simulink model "rebi"  (R2026a)
settings: Solver=ode1  StopTime=40  FixedStep=0.001  EnableMultiTasking=on
PostLoadFcn:
  | , if any(exist('dsrtsu_mdlpostloadfcn', 'file') == [2, 3, 6]), try dsrtsu_mdlpostloadfcn('Execute', bdroot); catch fprintf('Error in PostLoadFcn (dsrtsu_mdlpostloadfcn) for model "%s":\n %s\n', bdroot, lasterr); end, end,
values from neighbouring files (symbols this model uses):
  A = [0 1 ; -w0^2 -2*xhi*w0]    [integral_state_feedback_pole_placement.m]    (also in lqr_integral_control.m = [-2*xhi*omega0  -omega0^2  0     0           0)
  B = [0 ; k*w0]    [integral_state_feedback_pole_placement.m]    (also in lqr_integral_control.m = [Ke*omega0^2     Ke*omega0^2)
  C = [1 0]    [integral_state_feedback_pole_placement.m]    (also in lqr_integral_control.m = [0 1 0 0 0)
  Ki = K(:, n+1:n+p)    [lqr_integral_control.m]
  Kp = K(:, 1:n)    [lqr_integral_control.m]
settings Model: DSRTSU_INTERNAL_RTI_VER=370  DSRTSU_INTERNAL_RTI_TYPE=rti1104  Creator=eleve  LastModifiedBy=DevKumar
settings DataIOCC: SignalLoggingSaveFormat=ModelDataLogs
settings OptimizationCC: OptimizeBlockIOStorage=off  BufferReuse=off  ExpressionFolding=off  LocalBlockOutputs=off
settings DebuggingCC: UnderspecifiedInitializationDetection=Classic
settings HardwareCC: ProdEndianess=BigEndian  ProdHWDeviceType=Generic->Custom  TargetIntDivRoundTo=Zero  TargetEndianess=BigEndian  TargetHWDeviceType=Generic->Custom
settings RTWCC: SystemTargetFile=rti1104.tlc  MakeCommand=make_rti  TemplateMakefile=rti1104.tmf  Description=dSPACE DS1104 Hardware Platform
settings STFCustomTargetCC: SystemTargetFile=rti1104.tlc  MultiwordLength=2048.0  ParMdlRefBuildCompliant=on  CPPClassGenCompliant=on  TimeScaleFactorNonUI=OPTION_DISABLED  TimeScaleFactor=1.0  CCompilerOptimizationOptsPopup_=Default  ExecutionModeNonUI=RTSIM  TAStimulusEngineEnable=off  InitialSimState=RUN  AllowReservedHostServiceNums=off  ExecutionMode=real-time  AssertionMode=OFF  LoadAfterBuild=on  CCompilerEffectiveOptimizationOpts=-Ot -Oi -Or -Ox -D_INLINE  CCompilerOptimizationOptsNonUI=USE_DEFAULT  BoardNameNonUI=OPTION_DISABLED  LoadToFlash=off  TRCGenerateParamValues=off  LoadApplNonUI=ON  TRCApplySubsystemPermissions=off  PlatformSelectionPopup=Auto  TRCMaskParameters=off  TRCGenerateStates=off  TRCOnlyGlobals=off  TRCGenerateDerivatives=off  TRCGenerateLabels=on  TRCIsOmitVdOn=off  TRCGenerateVirtualBlocks=on
settings GRTTargetCC: ExtModeMexFile=noextcomm  CompOptLevelCompliant=off  ConcurrentExecutionCompliant=off  CombineOutputUpdateFcns=off  MatFileLogging=off  GRTInterface=on

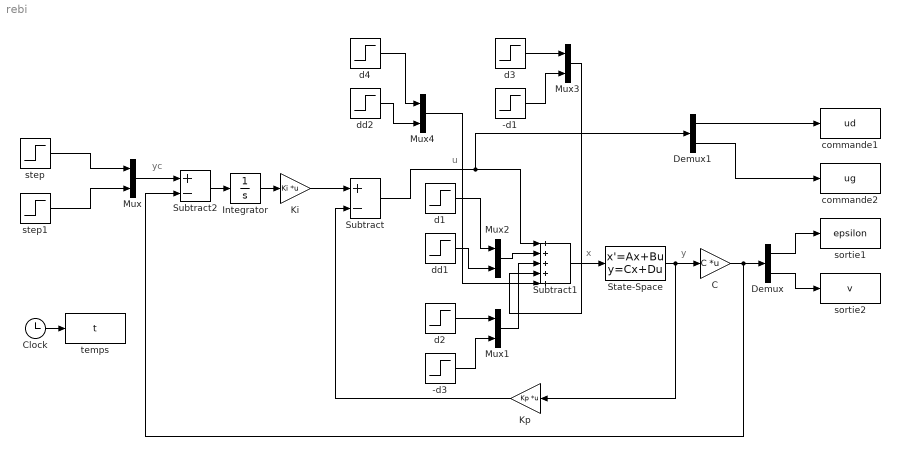
== system rebi ==
  note: u
  note: yc
  note: x
  note: y
  -d1 : Step  Time=11  FinalValue=5  SampleTime=0
  -d3 : Step  Time=10  FinalValue=-5  SampleTime=0
  C : Gain  Gain=C  Multiplication=Matrix(K*u) (u vector)
  Clock : Clock
  Demux : Demux  Outputs=2
  Demux1 : Demux  Outputs=2
  Integrator : Integrator
  Ki : Gain  Gain=Ki  Multiplication=Matrix(K*u) (u vector)
  Kp : Gain  Gain=Kp  Multiplication=Matrix(K*u) (u vector)
  Mux{,1..4} (5 alike) : Mux  Inputs=2
  State-Space : StateSpace  A=A  B=B  C=eye(5)  D=zeros(5,2)  InitialCondition=0
  Subtract : Sum  Inputs=+-
  Subtract1 : Sum  Inputs=+++++
  Subtract2 : Sum  Inputs=+-
  commande1 : ToWorkspace  VariableName=ud  SampleTime=-1
  commande2 : ToWorkspace  VariableName=ug  SampleTime=-1
  d1 : Step  Time=10  FinalValue=5  SampleTime=0
  d2 : Step  Time=10  FinalValue=5  SampleTime=0
  d3 : Step  Time=11  FinalValue=-5  SampleTime=0
  d4 : Step  Time=11  FinalValue=5  SampleTime=0
  dd1 : Step  Time=10  FinalValue=5  SampleTime=0
  dd2 : Step  Time=11  FinalValue=5  SampleTime=0
  sortie1 : ToWorkspace  VariableName=epsilon  SampleTime=-1
  sortie2 : ToWorkspace  VariableName=v  SampleTime=-1
  step : Step  FinalValue=pi/6  SampleTime=0
  step1 : Step  SampleTime=0
  temps : ToWorkspace  VariableName=t  SampleTime=-1
  wires:
  Subtract2/1 -> Integrator/1
  Integrator/1 -> Ki/1
  Ki/1 -> Subtract/1
  Kp/1 -> Subtract/2
  Subtract/1 -> Subtract1/1, Demux1/1
  State-Space/1 -> C/1, Kp/1
  Clock/1 -> temps/1
  C/1 -> Demux/1, Subtract2/2
  Demux/1 -> sortie1/1
  Demux/2 -> sortie2/1
  Demux1/1 -> commande1/1
  Demux1/2 -> commande2/1
  step/1 -> Mux/1
  step1/1 -> Mux/2
  Mux/1 -> Subtract2/1
  Subtract1/1 -> State-Space/1
  d1/1 -> Mux2/1
  dd1/1 -> Mux2/2
  Mux2/1 -> Subtract1/2
  d2/1 -> Mux1/1
  -d3/1 -> Mux1/2
  Mux1/1 -> Subtract1/3
  -d1/1 -> Mux3/2
  d3/1 -> Mux3/1
  Mux3/1 -> Subtract1/4
  dd2/1 -> Mux4/2
  Mux4/1 -> Subtract1/5
  d4/1 -> Mux4/1
